simulink model "model_v16Big_Rear_Braking_Haz"  (Simulink 7.6)
settings: Solver=ode45  StartTime=0.0  StopTime=10.0  RelTol=1e-3
Description:
  | <HiP-HOPS_Model_Parameters><ToolVersion><Name>Matlab</Name><Number>7.11.0.584 </Number></ToolVersion><RiskTime>10000</RiskTime><OptimisationParams></OptimisationParams><Hazards><Hazard><Name>No_Braking_Rear</Name><Description></Description><SafetyRequirement>4</SafetyRequirement><Causes><Cause><Probability></Probability><FailureLogic>Omission-Brake_Unit3.Add.Braking AND Omission-Brake_Unit4.Add.Braking</FailureLogic></Cause></Causes></Hazard><Hazard><Name>Value_Braking</Name><Description></Description><SafetyRequirement>4</SafetyRequirement><Causes><Cause><Probability></Probability><FailureLogic>Value-Brake_Unit3.Add.Braking AND Value-Brake_Unit4.Add.Braking</FailureLogic></Cause></Causes></Hazard></Hazards><AdvancedParameters></AdvancedParameters></HiP-HOPS_Model_Parameters>
settings Model: Creator=Asus  LastModifiedBy=André

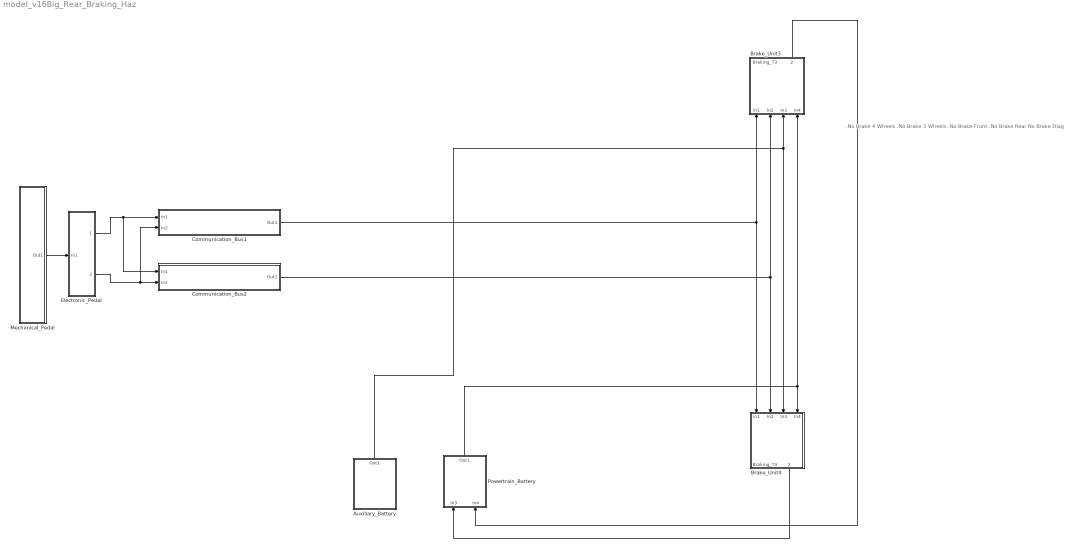
== system model_v16Big_Rear_Braking_Haz ==
  note: .No Brake 4 Wheels
      | .No Brake 3 Wheels
      | .No Brake Front
      | .No Brake Rear
      | No Brake Diag
  Auxiliary_Battery : Subsystem
  Brake_Unit3 : Subsystem
  Brake_Unit4 : Subsystem
  Communication_Bus1 : Subsystem
  Communication_Bus2 : Subsystem
  Electronic_Pedal : Subsystem
  Mechanical_Pedal : Subsystem
  Powertrain_Battery : Subsystem
  wires:
  Electronic_Pedal/1(Out1) -> Communication_Bus1/1(In1), Communication_Bus2/1(In1)
  Electronic_Pedal/2(Out2) -> Communication_Bus1/2(In2), Communication_Bus2/2(In2)
  Mechanical_Pedal/1(Out1) -> Electronic_Pedal/1(In1)
  Communication_Bus1/1(Out1) -> Brake_Unit3/1(In1), Brake_Unit4/1(In1)
  Communication_Bus2/1(Out1) -> Brake_Unit4/2(In2), Brake_Unit3/2(In2)
  Auxiliary_Battery/1(Out1) -> Brake_Unit3/3(In3), Brake_Unit4/3(In3)
  Powertrain_Battery/1(Out1) -> Brake_Unit4/4(In4), Brake_Unit3/4(In4)
  Brake_Unit4/2(Generated_Power4) -> Powertrain_Battery/1(In3)
  Brake_Unit3/2(Generated_Power3) -> Powertrain_Battery/2(In4)

== system model_v16Big_Rear_Braking_Haz/Auxiliary_Battery ==
  Out1 : Outport

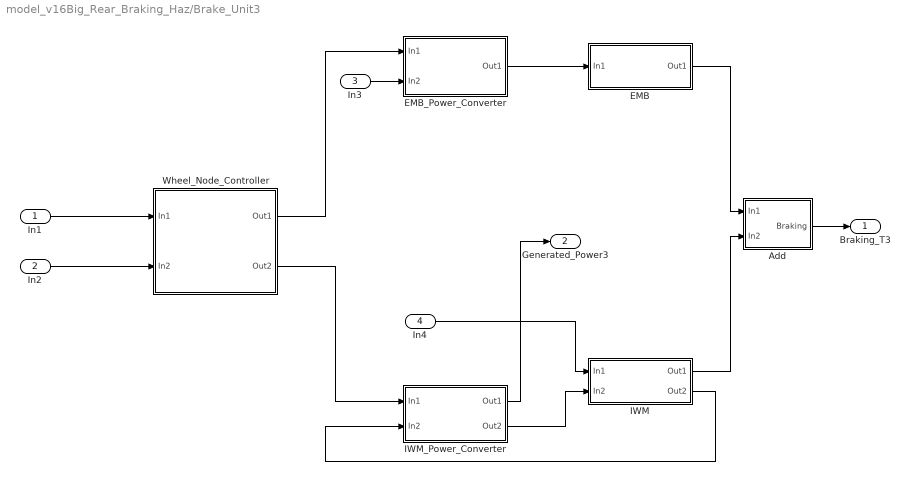
== system model_v16Big_Rear_Braking_Haz/Brake_Unit3 ==
  In1 : Inport
  In2 : Inport  Port=2
  In3 : Inport  Port=3
  In4 : Inport  Port=4
  Add : Subsystem
  EMB : Subsystem
  EMB_Power_Converter : Subsystem
  IWM : Subsystem
  IWM_Power_Converter : Subsystem
  Wheel_Node_Controller : Subsystem
  Braking_T3 : Outport
  Generated_Power3 : Outport  Port=2
  wires:
  EMB_Power_Converter/1(Out1) -> EMB/1(In1)
  Add/1(Braking) -> Braking_T3/1
  Wheel_Node_Controller/1(Out1) -> EMB_Power_Converter/1(In1)
  EMB/1(Out1) -> Add/1(In1)
  IWM/1(Out1) -> Add/2(In2)
  IWM/2(Out2) -> IWM_Power_Converter/2(In2)
  IWM_Power_Converter/2(Out2) -> IWM/2(In2)
  Wheel_Node_Controller/2(Out2) -> IWM_Power_Converter/1(In1)
  In1/1 -> Wheel_Node_Controller/1(In1)
  In2/1 -> Wheel_Node_Controller/2(In2)
  In3/1 -> EMB_Power_Converter/2(In2)
  IWM_Power_Converter/1(Out1) -> Generated_Power3/1
  In4/1 -> IWM/1(In1)

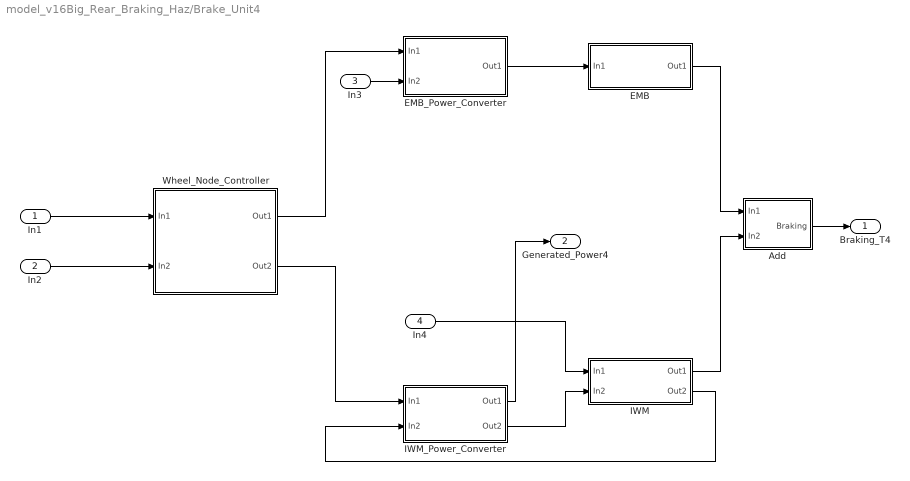
== system model_v16Big_Rear_Braking_Haz/Brake_Unit4 ==
  In1 : Inport
  In2 : Inport  Port=2
  In3 : Inport  Port=3
  In4 : Inport  Port=4
  Add : Subsystem
  EMB : Subsystem
  EMB_Power_Converter : Subsystem
  IWM : Subsystem
  IWM_Power_Converter : Subsystem
  Wheel_Node_Controller : Subsystem
  Braking_T4 : Outport
  Generated_Power4 : Outport  Port=2
  wires:
  EMB_Power_Converter/1(Out1) -> EMB/1(In1)
  Add/1(Braking) -> Braking_T4/1
  Wheel_Node_Controller/1(Out1) -> EMB_Power_Converter/1(In1)
  EMB/1(Out1) -> Add/1(In1)
  IWM/1(Out1) -> Add/2(In2)
  IWM/2(Out2) -> IWM_Power_Converter/2(In2)
  IWM_Power_Converter/2(Out2) -> IWM/2(In2)
  Wheel_Node_Controller/2(Out2) -> IWM_Power_Converter/1(In1)
  In1/1 -> Wheel_Node_Controller/1(In1)
  In2/1 -> Wheel_Node_Controller/2(In2)
  In3/1 -> EMB_Power_Converter/2(In2)
  IWM_Power_Converter/1(Out1) -> Generated_Power4/1
  In4/1 -> IWM/1(In1)

== system model_v16Big_Rear_Braking_Haz/Communication_Bus1 ==
  In1 : Inport
  In2 : Inport  Port=2
  Out1 : Outport

== system model_v16Big_Rear_Braking_Haz/Communication_Bus2 ==
  In1 : Inport
  In2 : Inport  Port=2
  Out1 : Outport

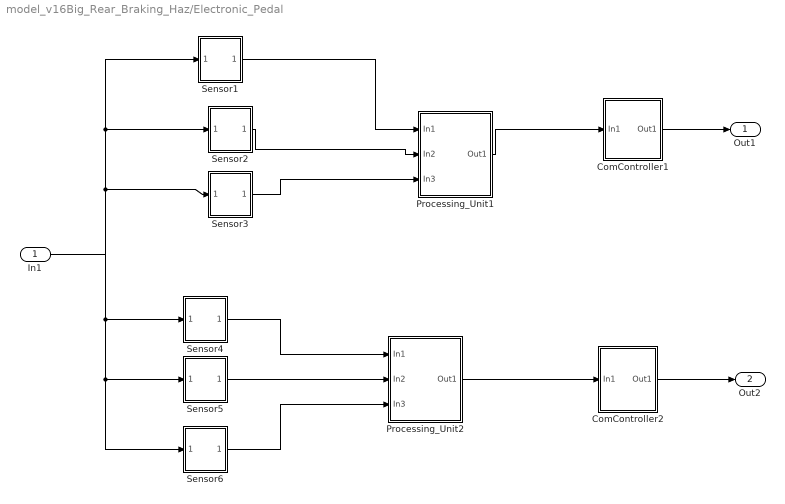
== system model_v16Big_Rear_Braking_Haz/Electronic_Pedal ==
  In1 : Inport
  ComController1 : Subsystem
  ComController2 : Subsystem
  Processing_Unit1 : Subsystem
  Processing_Unit2 : Subsystem
  Sensor1 : Subsystem
  Sensor2 : Subsystem
  Sensor3 : Subsystem
  Sensor4 : Subsystem
  Sensor5 : Subsystem
  Sensor6 : Subsystem
  Out1 : Outport
  Out2 : Outport  Port=2
  wires:
  In1/1 -> Sensor5/1(In1), Sensor6/1(In1), Sensor4/1(In1), Sensor1/1(In1), Sensor2/1(In1), Sensor3/1(In1)
  ComController1/1(Out1) -> Out1/1
  ComController2/1(Out1) -> Out2/1
  Sensor1/1(Out1) -> Processing_Unit1/1(In1)
  Sensor2/1(Out1) -> Processing_Unit1/2(In2)
  Sensor3/1(Out1) -> Processing_Unit1/3(In3)
  Processing_Unit1/1(Out1) -> ComController1/1(In1)
  Sensor4/1(Out1) -> Processing_Unit2/1(In1)
  Sensor5/1(Out1) -> Processing_Unit2/2(In2)
  Sensor6/1(Out1) -> Processing_Unit2/3(In3)
  Processing_Unit2/1(Out1) -> ComController2/1(In1)

== system model_v16Big_Rear_Braking_Haz/Mechanical_Pedal ==
  Out1 : Outport

== system model_v16Big_Rear_Braking_Haz/Powertrain_Battery ==
  In3 : Inport
  In4 : Inport  Port=2
  Out1 : Outport

== system model_v16Big_Rear_Braking_Haz/Brake_Unit3/Add ==
  In1 : Inport
  In2 : Inport  Port=2
  Braking : Outport

== system model_v16Big_Rear_Braking_Haz/Brake_Unit3/EMB ==
  In1 : Inport
  Out1 : Outport

== system model_v16Big_Rear_Braking_Haz/Brake_Unit3/EMB_Power_Converter ==
  In1 : Inport
  In2 : Inport  Port=2
  Out1 : Outport

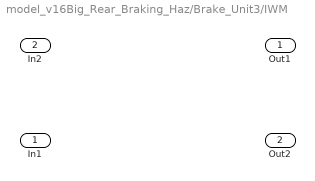
== system model_v16Big_Rear_Braking_Haz/Brake_Unit3/IWM ==
  In1 : Inport
  In2 : Inport  Port=2
  Out1 : Outport
  Out2 : Outport  Port=2

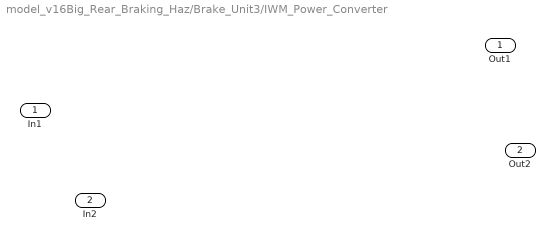
== system model_v16Big_Rear_Braking_Haz/Brake_Unit3/IWM_Power_Converter ==
  In1 : Inport
  In2 : Inport  Port=2
  Out1 : Outport
  Out2 : Outport  Port=2

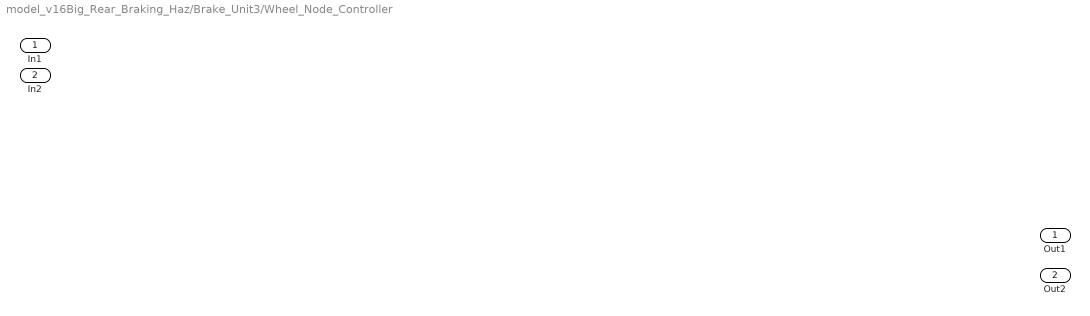
== system model_v16Big_Rear_Braking_Haz/Brake_Unit3/Wheel_Node_Controller ==
  In1 : Inport
  In2 : Inport  Port=2
  Out1 : Outport
  Out2 : Outport  Port=2

== system model_v16Big_Rear_Braking_Haz/Brake_Unit4/Add ==
  In1 : Inport
  In2 : Inport  Port=2
  Braking : Outport

== system model_v16Big_Rear_Braking_Haz/Brake_Unit4/EMB ==
  In1 : Inport
  Out1 : Outport

== system model_v16Big_Rear_Braking_Haz/Brake_Unit4/EMB_Power_Converter ==
  In1 : Inport
  In2 : Inport  Port=2
  Out1 : Outport

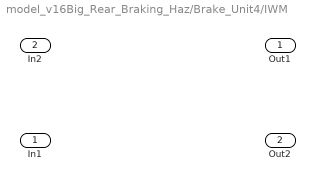
== system model_v16Big_Rear_Braking_Haz/Brake_Unit4/IWM ==
  In1 : Inport
  In2 : Inport  Port=2
  Out1 : Outport
  Out2 : Outport  Port=2

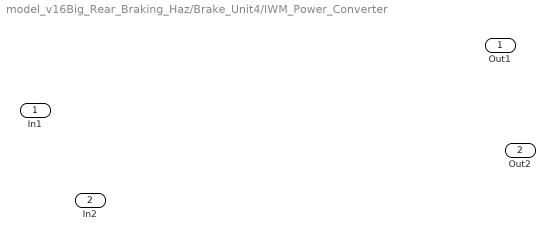
== system model_v16Big_Rear_Braking_Haz/Brake_Unit4/IWM_Power_Converter ==
  In1 : Inport
  In2 : Inport  Port=2
  Out1 : Outport
  Out2 : Outport  Port=2

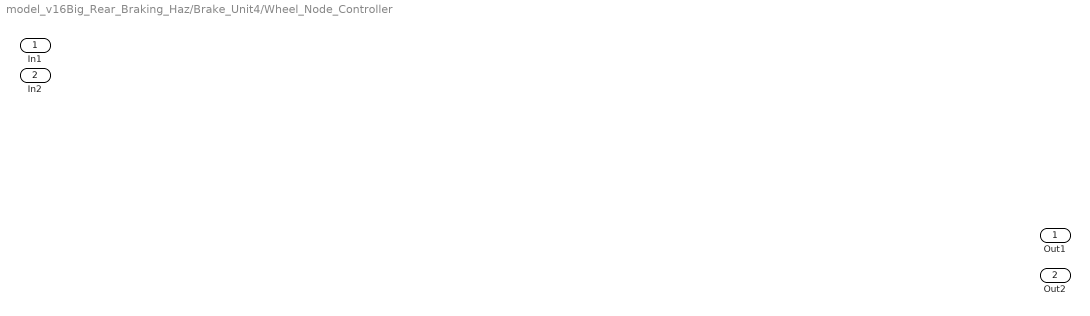
== system model_v16Big_Rear_Braking_Haz/Brake_Unit4/Wheel_Node_Controller ==
  In1 : Inport
  In2 : Inport  Port=2
  Out1 : Outport
  Out2 : Outport  Port=2

== system model_v16Big_Rear_Braking_Haz/Electronic_Pedal/ComController1 ==
  In1 : Inport
  Out1 : Outport

== system model_v16Big_Rear_Braking_Haz/Electronic_Pedal/ComController2 ==
  In1 : Inport
  Out1 : Outport

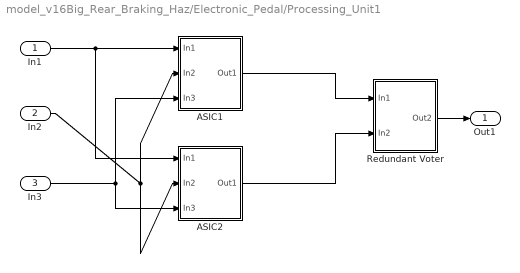
== system model_v16Big_Rear_Braking_Haz/Electronic_Pedal/Processing_Unit1 ==
  In1 : Inport
  In2 : Inport  Port=2
  In3 : Inport  Port=3
  ASIC1 : Subsystem
  ASIC2 : Subsystem
  Redundant Voter : Subsystem
  Out1 : Outport
  wires:
  ASIC1/1(Out1) -> Redundant Voter/1(In1)
  ASIC2/1(Out1) -> Redundant Voter/2(In2)
  In1/1 -> ASIC1/1(In1), ASIC2/1(In1)
  In2/1 -> ASIC2/2(In2), ASIC1/2(In2)
  Redundant Voter/1(Out2) -> Out1/1
  In3/1 -> ASIC1/3(In3), ASIC2/3(In3)

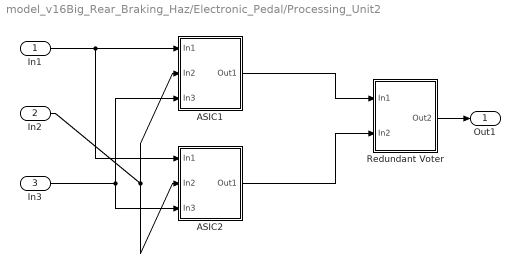
== system model_v16Big_Rear_Braking_Haz/Electronic_Pedal/Processing_Unit2 ==
  In1 : Inport
  In2 : Inport  Port=2
  In3 : Inport  Port=3
  ASIC1 : Subsystem
  ASIC2 : Subsystem
  Redundant Voter : Subsystem
  Out1 : Outport
  wires:
  ASIC1/1(Out1) -> Redundant Voter/1(In1)
  ASIC2/1(Out1) -> Redundant Voter/2(In2)
  In1/1 -> ASIC1/1(In1), ASIC2/1(In1)
  In2/1 -> ASIC2/2(In2), ASIC1/2(In2)
  Redundant Voter/1(Out2) -> Out1/1
  In3/1 -> ASIC1/3(In3), ASIC2/3(In3)

== system model_v16Big_Rear_Braking_Haz/Electronic_Pedal/Sensor1 ==
  In1 : Inport
  Out1 : Outport

== system model_v16Big_Rear_Braking_Haz/Electronic_Pedal/Sensor2 ==
  In1 : Inport
  Out1 : Outport

== system model_v16Big_Rear_Braking_Haz/Electronic_Pedal/Sensor3 ==
  In1 : Inport
  Out1 : Outport

== system model_v16Big_Rear_Braking_Haz/Electronic_Pedal/Sensor4 ==
  In1 : Inport
  Out1 : Outport

== system model_v16Big_Rear_Braking_Haz/Electronic_Pedal/Sensor5 ==
  In1 : Inport
  Out1 : Outport

== system model_v16Big_Rear_Braking_Haz/Electronic_Pedal/Sensor6 ==
  In1 : Inport
  Out1 : Outport

== system model_v16Big_Rear_Braking_Haz/Electronic_Pedal/Processing_Unit1/ASIC1 ==
  In1 : Inport
  In2 : Inport  Port=2
  In3 : Inport  Port=3
  Out1 : Outport

== system model_v16Big_Rear_Braking_Haz/Electronic_Pedal/Processing_Unit1/ASIC2 ==
  In1 : Inport
  In2 : Inport  Port=2
  In3 : Inport  Port=3
  Out1 : Outport

== system model_v16Big_Rear_Braking_Haz/Electronic_Pedal/Processing_Unit1/Redundant Voter ==
  In1 : Inport
  In2 : Inport  Port=2
  Out2 : Outport

== system model_v16Big_Rear_Braking_Haz/Electronic_Pedal/Processing_Unit2/ASIC1 ==
  In1 : Inport
  In2 : Inport  Port=2
  In3 : Inport  Port=3
  Out1 : Outport

== system model_v16Big_Rear_Braking_Haz/Electronic_Pedal/Processing_Unit2/ASIC2 ==
  In1 : Inport
  In2 : Inport  Port=2
  In3 : Inport  Port=3
  Out1 : Outport

== system model_v16Big_Rear_Braking_Haz/Electronic_Pedal/Processing_Unit2/Redundant Voter ==
  In1 : Inport
  In2 : Inport  Port=2
  Out2 : Outport
